simulink model "VGA_Interface"  (R2019b)
settings: Solver=VariableStepAuto  StartTime=0.0  StopTime=10.0  RelTol=1e-3
libraries: hdlsllib x24, simulink x20
settings Model: Creator=douglas.th  LastModifiedBy=Aaditya
settings DataIOCC: ReturnWorkspaceOutputs=off
settings OptimizationCC: BlockReduction=off  ConditionallyExecuteInputs=off  DefaultParameterBehavior=Inlined
settings DebuggingCC: AlgebraicLoopMsg=error  ArithmeticOperatorsInVariantConditions=warning
settings HardwareCC: ProdBitPerPointer=32  ProdBitPerSizeT=32  ProdBitPerPtrDiffT=32  ProdLargestAtomicFloat=None  ProdIntDivRoundTo=Undefined  ProdEndianess=Unspecified  ProdWordSize=32  ProdHWDeviceType=ASIC/FPGA->ASIC/FPGA  TargetBitPerPointer=64  TargetBitPerSizeT=64  TargetBitPerPtrDiffT=64  TargetLongLongMode=on  TargetIntDivRoundTo=Zero  TargetEndianess=LittleEndian  TargetWordSize=64  TargetHWDeviceType=Custom Processor->MATLAB Host Computer  ProdEqTarget=off
settings SFSimCC: SimUseLocalCustomCode=off  CustomCodeUndefinedFunction=UseInterfaceOnly
settings RTWCC: RTWUseLocalCustomCode=off

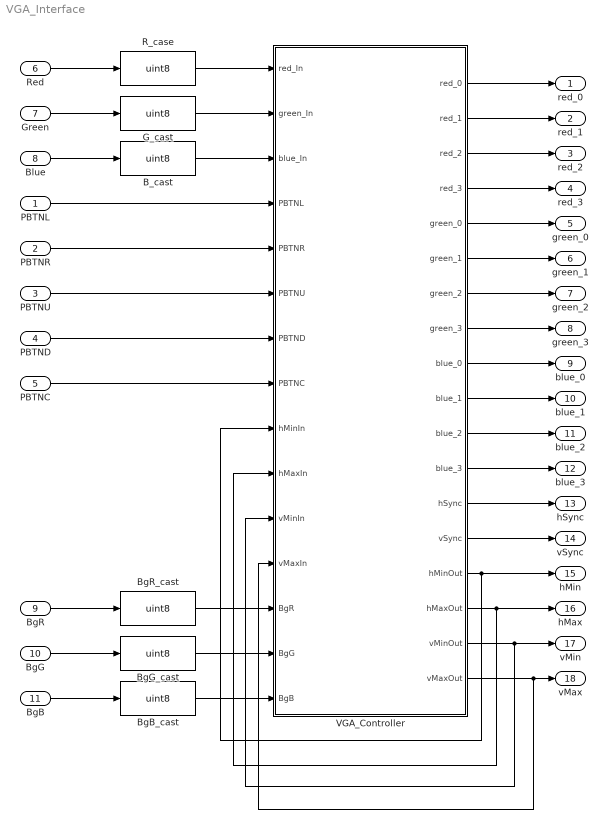
== system VGA_Interface ==
  PBTNL : Inport
  PBTNR : Inport  Port=2
  PBTNU : Inport  Port=3
  PBTND : Inport  Port=4
  PBTNC : Inport  Port=5
  Red : Inport  Port=6
  Green : Inport  Port=7
  Blue : Inport  Port=8
  BgR : Inport  Port=9
  BgG : Inport  Port=10
  BgB : Inport  Port=11
  B_cast : DataTypeConversion  OutDataTypeStr=uint8
  BgB_cast : DataTypeConversion  OutDataTypeStr=uint8
  BgG_cast : DataTypeConversion  OutDataTypeStr=uint8
  BgR_cast : DataTypeConversion  OutDataTypeStr=uint8
  G_cast : DataTypeConversion  OutDataTypeStr=uint8
  R_case : DataTypeConversion  OutDataTypeStr=uint8
  VGA_Controller : Subsystem
  red_0 : Outport  VectorParamsAs1DForOutWhenUnconnected=off
  red_1 : Outport  Port=2  VectorParamsAs1DForOutWhenUnconnected=off
  red_2 : Outport  Port=3  VectorParamsAs1DForOutWhenUnconnected=off
  red_3 : Outport  Port=4  VectorParamsAs1DForOutWhenUnconnected=off
  green_0 : Outport  Port=5  VectorParamsAs1DForOutWhenUnconnected=off
  green_1 : Outport  Port=6  VectorParamsAs1DForOutWhenUnconnected=off
  green_2 : Outport  Port=7  VectorParamsAs1DForOutWhenUnconnected=off
  green_3 : Outport  Port=8  VectorParamsAs1DForOutWhenUnconnected=off
  blue_0 : Outport  Port=9  VectorParamsAs1DForOutWhenUnconnected=off
  blue_1 : Outport  Port=10  VectorParamsAs1DForOutWhenUnconnected=off
  blue_2 : Outport  Port=11  VectorParamsAs1DForOutWhenUnconnected=off
  blue_3 : Outport  Port=12  VectorParamsAs1DForOutWhenUnconnected=off
  hSync : Outport  Port=13  VectorParamsAs1DForOutWhenUnconnected=off
  vSync : Outport  Port=14  VectorParamsAs1DForOutWhenUnconnected=off
  hMin : Outport  Port=15  VectorParamsAs1DForOutWhenUnconnected=off
  hMax : Outport  Port=16  VectorParamsAs1DForOutWhenUnconnected=off
  vMin : Outport  Port=17  VectorParamsAs1DForOutWhenUnconnected=off
  vMax : Outport  Port=18  VectorParamsAs1DForOutWhenUnconnected=off
  wires:
  VGA_Controller/1(red_0) -> red_0/1
  VGA_Controller/2(red_1) -> red_1/1
  VGA_Controller/3(red_2) -> red_2/1
  VGA_Controller/4(red_3) -> red_3/1
  VGA_Controller/5(green_0) -> green_0/1
  VGA_Controller/6(green_1) -> green_1/1
  VGA_Controller/7(green_2) -> green_2/1
  VGA_Controller/8(green_3) -> green_3/1
  VGA_Controller/9(blue_0) -> blue_0/1
  VGA_Controller/10(blue_1) -> blue_1/1
  VGA_Controller/11(blue_2) -> blue_2/1
  VGA_Controller/12(blue_3) -> blue_3/1
  VGA_Controller/14(vSync) -> vSync/1
  VGA_Controller/13(hSync) -> hSync/1
  Blue/1 -> B_cast/1
  G_cast/1 -> VGA_Controller/2(green_In)
  R_case/1 -> VGA_Controller/1(red_In)
  PBTNL/1 -> VGA_Controller/4(PBTNL)
  PBTNR/1 -> VGA_Controller/5(PBTNR)
  PBTNU/1 -> VGA_Controller/6(PBTNU)
  PBTND/1 -> VGA_Controller/7(PBTND)
  PBTNC/1 -> VGA_Controller/8(PBTNC)
  Red/1 -> R_case/1
  Green/1 -> G_cast/1
  B_cast/1 -> VGA_Controller/3(blue_In)
  VGA_Controller/16(hMaxOut) -> hMax/1, VGA_Controller/10(hMaxIn)
  VGA_Controller/15(hMinOut) -> VGA_Controller/9(hMinIn), hMin/1
  VGA_Controller/18(vMaxOut) -> VGA_Controller/12(vMaxIn), vMax/1
  VGA_Controller/17(vMinOut) -> vMin/1, VGA_Controller/11(vMinIn)
  BgB/1 -> BgB_cast/1
  BgB_cast/1 -> VGA_Controller/15(BgB)
  BgR/1 -> BgR_cast/1
  BgR_cast/1 -> VGA_Controller/13(BgR)
  BgG_cast/1 -> VGA_Controller/14(BgG)
  BgG/1 -> BgG_cast/1

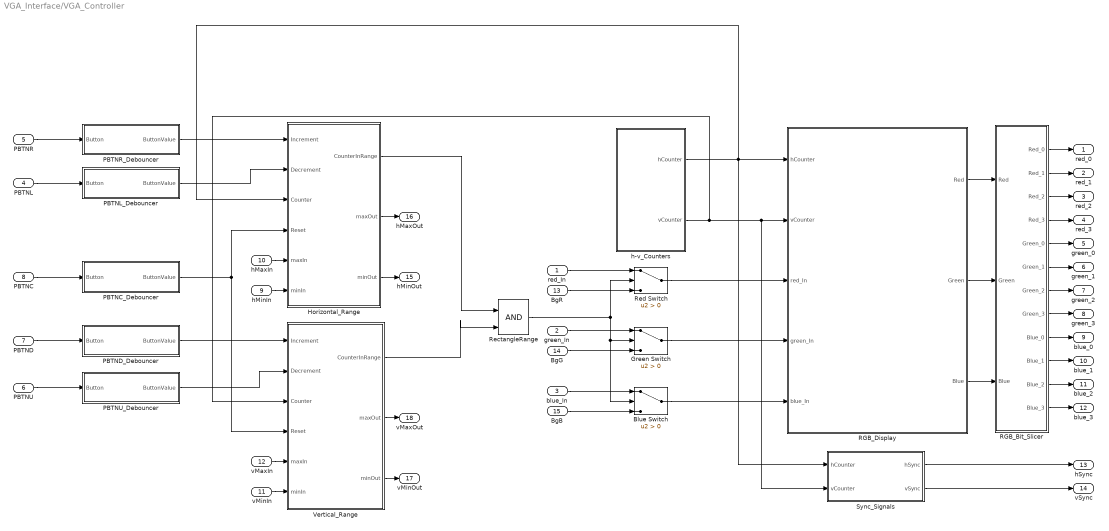
== system VGA_Interface/VGA_Controller ==
  red_In : Inport  OutDataTypeStr=uint8
  green_In : Inport  Port=2  OutDataTypeStr=uint8
  blue_In : Inport  Port=3  OutDataTypeStr=uint8
  PBTNL : Inport  Port=4  OutDataTypeStr=boolean
  PBTNR : Inport  Port=5  OutDataTypeStr=boolean
  PBTNU : Inport  Port=6  OutDataTypeStr=boolean
  PBTND : Inport  Port=7  OutDataTypeStr=boolean
  PBTNC : Inport  Port=8  OutDataTypeStr=boolean
  hMinIn : Inport  Port=9
  hMaxIn : Inport  Port=10
  vMinIn : Inport  Port=11
  vMaxIn : Inport  Port=12
  BgR : Inport  Port=13
  BgG : Inport  Port=14
  BgB : Inport  Port=15
  Blue Switch : Switch  Criteria=u2 > Threshold
  Green Switch : Switch  Criteria=u2 > Threshold
  Horizontal_Range : Subsystem
  PBTNC_Debouncer : Subsystem
  PBTND_Debouncer : Subsystem
  PBTNL_Debouncer : Subsystem
  PBTNR_Debouncer : Subsystem
  PBTNU_Debouncer : Subsystem
  RGB_Bit_Slicer : Subsystem
  RGB_Display : Subsystem
  RectangleRange : Logic  IconShape=distinctive  AllPortsSameDT=off  OutDataTypeStr=boolean
  Red Switch : Switch  Criteria=u2 > Threshold
  Sync_Signals : Subsystem
  Vertical_Range : Subsystem
  "h-v_Counters " : Subsystem
  red_0 : Outport  VectorParamsAs1DForOutWhenUnconnected=off
  red_1 : Outport  Port=2  VectorParamsAs1DForOutWhenUnconnected=off
  red_2 : Outport  Port=3  VectorParamsAs1DForOutWhenUnconnected=off
  red_3 : Outport  Port=4  VectorParamsAs1DForOutWhenUnconnected=off
  green_0 : Outport  Port=5  VectorParamsAs1DForOutWhenUnconnected=off
  green_1 : Outport  Port=6  VectorParamsAs1DForOutWhenUnconnected=off
  green_2 : Outport  Port=7  VectorParamsAs1DForOutWhenUnconnected=off
  green_3 : Outport  Port=8  VectorParamsAs1DForOutWhenUnconnected=off
  blue_0 : Outport  Port=9  VectorParamsAs1DForOutWhenUnconnected=off
  blue_1 : Outport  Port=10  VectorParamsAs1DForOutWhenUnconnected=off
  blue_2 : Outport  Port=11  VectorParamsAs1DForOutWhenUnconnected=off
  blue_3 : Outport  Port=12  VectorParamsAs1DForOutWhenUnconnected=off
  hSync : Outport  Port=13  VectorParamsAs1DForOutWhenUnconnected=off
  vSync : Outport  Port=14  VectorParamsAs1DForOutWhenUnconnected=off
  hMinOut : Outport  Port=15  VectorParamsAs1DForOutWhenUnconnected=off
  hMaxOut : Outport  Port=16  VectorParamsAs1DForOutWhenUnconnected=off
  vMinOut : Outport  Port=17  VectorParamsAs1DForOutWhenUnconnected=off
  vMaxOut : Outport  Port=18  VectorParamsAs1DForOutWhenUnconnected=off
  wires:
  RGB_Display/1(Red) -> RGB_Bit_Slicer/1(Red)
  RGB_Bit_Slicer/4(Red_3) -> red_3/1
  RGB_Display/2(Green) -> RGB_Bit_Slicer/2(Green)
  Sync_Signals/2(vSync) -> vSync/1
  RGB_Bit_Slicer/6(Green_1) -> green_1/1
  RGB_Bit_Slicer/1(Red_0) -> red_0/1
  RGB_Display/3(Blue) -> RGB_Bit_Slicer/3(Blue)
  Sync_Signals/1(hSync) -> hSync/1
  RGB_Bit_Slicer/3(Red_2) -> red_2/1
  RGB_Bit_Slicer/2(Red_1) -> red_1/1
  RGB_Bit_Slicer/5(Green_0) -> green_0/1
  RGB_Bit_Slicer/7(Green_2) -> green_2/1
  RGB_Bit_Slicer/8(Green_3) -> green_3/1
  RGB_Bit_Slicer/9(Blue_0) -> blue_0/1
  RGB_Bit_Slicer/10(Blue_1) -> blue_1/1
  RGB_Bit_Slicer/11(Blue_2) -> blue_2/1
  RGB_Bit_Slicer/12(Blue_3) -> blue_3/1
  red_In/1 -> Red Switch/1
  blue_In/1 -> Blue Switch/1
  green_In/1 -> Green Switch/1
  "h-v_Counters "/1(hCounter) -> RGB_Display/1(hCounter), Sync_Signals/1(hCounter), Horizontal_Range/3(Counter)
  Red Switch/1 -> RGB_Display/3(red_In)
  Green Switch/1 -> RGB_Display/4(green_In)
  Blue Switch/1 -> RGB_Display/5(blue_In)
  PBTNL/1 -> PBTNL_Debouncer/1(Button)
  PBTNR/1 -> PBTNR_Debouncer/1(Button)
  PBTNU/1 -> PBTNU_Debouncer/1(Button)
  PBTNC/1 -> PBTNC_Debouncer/1(Button)
  PBTNC_Debouncer/1(ButtonValue) -> Vertical_Range/4(Reset), Horizontal_Range/4(Reset)
  Horizontal_Range/1(CounterInRange) -> RectangleRange/1
  Vertical_Range/1(CounterInRange) -> RectangleRange/2
  RectangleRange/1 -> Red Switch/2, Blue Switch/2, Green Switch/2
  "h-v_Counters "/2(vCounter) -> Vertical_Range/3(Counter), RGB_Display/2(vCounter), Sync_Signals/2(vCounter)
  vMaxIn/1 -> Vertical_Range/5(maxIn)
  vMinIn/1 -> Vertical_Range/6(minIn)
  hMinIn/1 -> Horizontal_Range/6(minIn)
  hMaxIn/1 -> Horizontal_Range/5(maxIn)
  Horizontal_Range/3(minOut) -> hMinOut/1
  Horizontal_Range/2(maxOut) -> hMaxOut/1
  Vertical_Range/2(maxOut) -> vMaxOut/1
  Vertical_Range/3(minOut) -> vMinOut/1
  PBTNU_Debouncer/1(ButtonValue) -> Vertical_Range/2(Decrement)
  PBTNR_Debouncer/1(ButtonValue) -> Horizontal_Range/1(Increment)
  PBTNL_Debouncer/1(ButtonValue) -> Horizontal_Range/2(Decrement)
  PBTND_Debouncer/1(ButtonValue) -> Vertical_Range/1(Increment)
  PBTND/1 -> PBTND_Debouncer/1(Button)
  BgR/1 -> Red Switch/3
  BgG/1 -> Green Switch/3
  BgB/1 -> Blue Switch/3

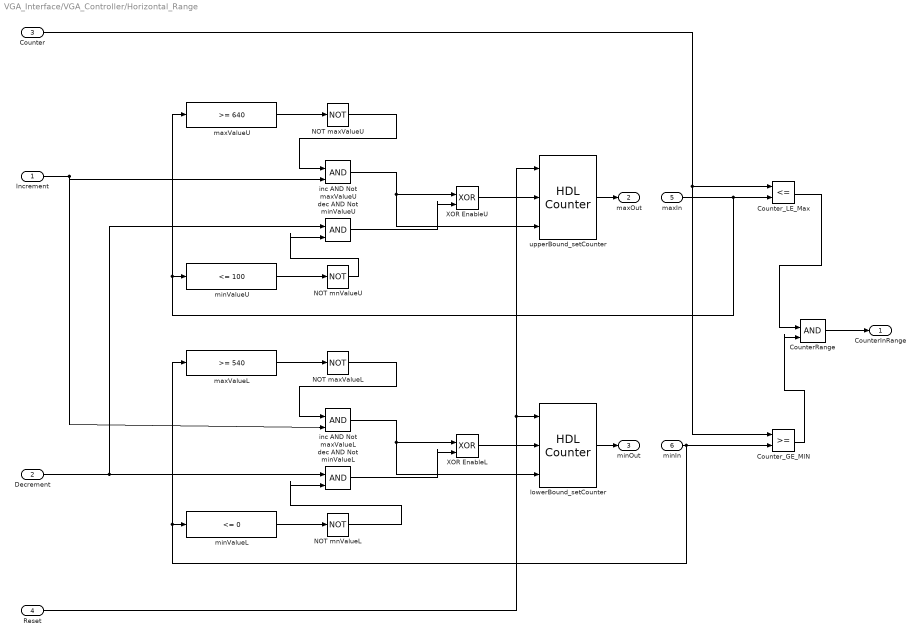
== system VGA_Interface/VGA_Controller/Horizontal_Range ==
  Increment : Inport
  Decrement : Inport  Port=2
  Counter : Inport  Port=3
  Reset : Inport  Port=4
  maxIn : Inport  Port=5  OutDataTypeStr=uint16
  minIn : Inport  Port=6  OutDataTypeStr=uint16
  CounterRange : Logic  IconShape=distinctive  AllPortsSameDT=off  OutDataTypeStr=boolean
  Counter_GE_MIN : RelationalOperator  OutDataTypeStr=boolean  RndMeth=Simplest
  Counter_LE_Max : RelationalOperator  Operator=<=  OutDataTypeStr=boolean  RndMeth=Simplest
  NOT maxValueL : Logic  Operator=NOT  IconShape=distinctive  AllPortsSameDT=off  OutDataTypeStr=boolean
  NOT maxValueU : Logic  Operator=NOT  IconShape=distinctive  AllPortsSameDT=off  OutDataTypeStr=boolean
  NOT mnValueL : Logic  Operator=NOT  IconShape=distinctive  AllPortsSameDT=off  OutDataTypeStr=boolean
  NOT mnValueU : Logic  Operator=NOT  IconShape=distinctive  AllPortsSameDT=off  OutDataTypeStr=boolean
  XOR EnableL : Logic  Operator=XOR  IconShape=distinctive  AllPortsSameDT=off  OutDataTypeStr=boolean
  XOR EnableU : Logic  Operator=XOR  IconShape=distinctive  AllPortsSameDT=off  OutDataTypeStr=boolean
  dec AND Not minValueL : Logic  IconShape=distinctive  AllPortsSameDT=off  OutDataTypeStr=boolean
  dec AND Not minValueU : Logic  IconShape=distinctive  AllPortsSameDT=off  OutDataTypeStr=boolean
  inc AND Not maxValueL : Logic  IconShape=distinctive  AllPortsSameDT=off  OutDataTypeStr=boolean
  inc AND Not maxValueU : Logic  IconShape=distinctive  AllPortsSameDT=off  OutDataTypeStr=boolean
  lowerBound_setCounter : hdlsllib/Sources/HDL Counter  CountType=Count limited  CountInit=0  CountStep=1  CountMax=540  CountFromType=Specify  CountFrom=0  CountResetPort=on  CountLoadPort=off  CountEnbPort=on  CountDirPort=on  CountDataType=Unsigned  CountWordLen=16  CountFracLen=0  CountSampTime=1
      settings: SourceProductBaseCode=HD
  maxValueL : simulink/Logic and Bit Operations/Compare To Constant  relop=>=  const=540  OutDataTypeStr=boolean
  maxValueU : simulink/Logic and Bit Operations/Compare To Constant  relop=>=  const=640  OutDataTypeStr=boolean
  minValueL : simulink/Logic and Bit Operations/Compare To Constant  relop=<=  const=0  OutDataTypeStr=boolean
  minValueU : simulink/Logic and Bit Operations/Compare To Constant  relop=<=  const=100  OutDataTypeStr=boolean
  upperBound_setCounter : hdlsllib/Sources/HDL Counter  CountType=Count limited  CountInit=100  CountStep=1  CountMax=640  CountFromType=Specify  CountFrom=100  CountResetPort=on  CountLoadPort=off  CountEnbPort=on  CountDirPort=on  CountDataType=Unsigned  CountWordLen=16  CountFracLen=0  CountSampTime=1
      settings: SourceProductBaseCode=HD
  CounterInRange : Outport  VectorParamsAs1DForOutWhenUnconnected=off
  maxOut : Outport  Port=2  OutDataTypeStr=uint16  VectorParamsAs1DForOutWhenUnconnected=off
  minOut : Outport  Port=3  OutDataTypeStr=uint16  VectorParamsAs1DForOutWhenUnconnected=off
  wires:
  inc AND Not maxValueU/1 -> XOR EnableU/1, upperBound_setCounter/3
  XOR EnableU/1 -> upperBound_setCounter/2
  minValueU/1 -> NOT mnValueU/1
  upperBound_setCounter/1 -> maxOut/1
  NOT maxValueU/1 -> inc AND Not maxValueU/1
  NOT mnValueU/1 -> dec AND Not minValueU/2
  maxValueU/1 -> NOT maxValueU/1
  dec AND Not minValueU/1 -> XOR EnableU/2
  Counter_LE_Max/1 -> CounterRange/1
  dec AND Not minValueL/1 -> XOR EnableL/2
  inc AND Not maxValueL/1 -> XOR EnableL/1, lowerBound_setCounter/3
  minValueL/1 -> NOT mnValueL/1
  NOT mnValueL/1 -> dec AND Not minValueL/2
  XOR EnableL/1 -> lowerBound_setCounter/2
  lowerBound_setCounter/1 -> minOut/1
  maxValueL/1 -> NOT maxValueL/1
  Counter/1 -> Counter_LE_Max/1, Counter_GE_MIN/1
  NOT maxValueL/1 -> inc AND Not maxValueL/1
  Counter_GE_MIN/1 -> CounterRange/2
  CounterRange/1 -> CounterInRange/1
  Decrement/1 -> dec AND Not minValueL/1, dec AND Not minValueU/1
  Increment/1 -> inc AND Not maxValueU/2, inc AND Not maxValueL/2
  Reset/1 -> upperBound_setCounter/1, lowerBound_setCounter/1
  maxIn/1 -> minValueU/1, maxValueU/1, Counter_LE_Max/2
  minIn/1 -> maxValueL/1, minValueL/1, Counter_GE_MIN/2

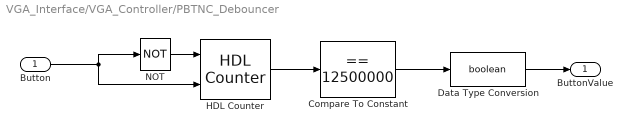
== system VGA_Interface/VGA_Controller/PBTNC_Debouncer ==
  Button : Inport
  Compare To Constant : simulink/Logic and Bit Operations/Compare To Constant  relop===  const=12500000  OutDataTypeStr=boolean
  Data Type Conversion : DataTypeConversion  OutDataTypeStr=boolean
  HDL Counter : hdlsllib/Sources/HDL Counter  CountType=Count limited  CountInit=0  CountStep=1  CountMax=50000000  CountFromType=Initial value  CountFrom=0  CountResetPort=on  CountLoadPort=off  CountEnbPort=on  CountDirPort=off  CountDataType=Unsigned  CountWordLen=32  CountFracLen=0  CountSampTime=1
      settings: SourceProductName=Simulink
  NOT : Logic  Operator=NOT  IconShape=distinctive  AllPortsSameDT=off  OutDataTypeStr=boolean
  ButtonValue : Outport  VectorParamsAs1DForOutWhenUnconnected=off
  wires:
  HDL Counter/1 -> Compare To Constant/1
  Compare To Constant/1 -> Data Type Conversion/1
  NOT/1 -> HDL Counter/1
  Button/1 -> HDL Counter/2, NOT/1
  Data Type Conversion/1 -> ButtonValue/1

== system VGA_Interface/VGA_Controller/PBTND_Debouncer ==
  Button : Inport
  Compare To Constant : simulink/Logic and Bit Operations/Compare To Constant  relop===  const=150000  OutDataTypeStr=boolean
  Data Type Conversion : DataTypeConversion  OutDataTypeStr=boolean
  HDL Counter : hdlsllib/Sources/HDL Counter  CountType=Count limited  CountInit=0  CountStep=1  CountMax=150000  CountFromType=Initial value  CountFrom=0  CountResetPort=on  CountLoadPort=off  CountEnbPort=on  CountDirPort=off  CountDataType=Unsigned  CountWordLen=32  CountFracLen=0  CountSampTime=1
      settings: SourceProductName=Simulink
  NOT : Logic  Operator=NOT  IconShape=distinctive  AllPortsSameDT=off  OutDataTypeStr=boolean
  ButtonValue : Outport  VectorParamsAs1DForOutWhenUnconnected=off
  wires:
  NOT/1 -> HDL Counter/1
  Button/1 -> HDL Counter/2, NOT/1
  Compare To Constant/1 -> Data Type Conversion/1
  HDL Counter/1 -> Compare To Constant/1
  Data Type Conversion/1 -> ButtonValue/1

== system VGA_Interface/VGA_Controller/PBTNL_Debouncer ==
  Button : Inport
  Compare To Constant : simulink/Logic and Bit Operations/Compare To Constant  relop===  const=150000  OutDataTypeStr=boolean
  Data Type Conversion : DataTypeConversion  OutDataTypeStr=boolean
  HDL Counter : hdlsllib/Sources/HDL Counter  CountType=Count limited  CountInit=0  CountStep=1  CountMax=150000  CountFromType=Initial value  CountFrom=0  CountResetPort=on  CountLoadPort=off  CountEnbPort=on  CountDirPort=off  CountDataType=Unsigned  CountWordLen=32  CountFracLen=0  CountSampTime=1
      settings: SourceProductName=Simulink
  NOT : Logic  Operator=NOT  IconShape=distinctive  AllPortsSameDT=off  OutDataTypeStr=boolean
  ButtonValue : Outport  VectorParamsAs1DForOutWhenUnconnected=off
  wires:
  NOT/1 -> HDL Counter/1
  Button/1 -> HDL Counter/2, NOT/1
  Compare To Constant/1 -> Data Type Conversion/1
  HDL Counter/1 -> Compare To Constant/1
  Data Type Conversion/1 -> ButtonValue/1

== system VGA_Interface/VGA_Controller/PBTNR_Debouncer ==
  Button : Inport
  Compare To Constant : simulink/Logic and Bit Operations/Compare To Constant  relop===  const=150000  OutDataTypeStr=boolean
  Data Type Conversion : DataTypeConversion  OutDataTypeStr=boolean
  HDL Counter : hdlsllib/Sources/HDL Counter  CountType=Count limited  CountInit=0  CountStep=1  CountMax=150000  CountFromType=Initial value  CountFrom=0  CountResetPort=on  CountLoadPort=off  CountEnbPort=on  CountDirPort=off  CountDataType=Unsigned  CountWordLen=32  CountFracLen=0  CountSampTime=1
      settings: SourceProductName=Simulink
  NOT : Logic  Operator=NOT  IconShape=distinctive  AllPortsSameDT=off  OutDataTypeStr=boolean
  ButtonValue : Outport  VectorParamsAs1DForOutWhenUnconnected=off
  wires:
  Button/1 -> HDL Counter/2, NOT/1
  Data Type Conversion/1 -> ButtonValue/1
  Compare To Constant/1 -> Data Type Conversion/1
  NOT/1 -> HDL Counter/1
  HDL Counter/1 -> Compare To Constant/1

== system VGA_Interface/VGA_Controller/PBTNU_Debouncer ==
  Button : Inport
  Compare To Constant : simulink/Logic and Bit Operations/Compare To Constant  relop===  const=150000  OutDataTypeStr=boolean
  Data Type Conversion : DataTypeConversion  OutDataTypeStr=boolean
  HDL Counter : hdlsllib/Sources/HDL Counter  CountType=Count limited  CountInit=0  CountStep=1  CountMax=150000  CountFromType=Initial value  CountFrom=0  CountResetPort=on  CountLoadPort=off  CountEnbPort=on  CountDirPort=off  CountDataType=Unsigned  CountWordLen=32  CountFracLen=0  CountSampTime=1
      settings: SourceProductName=Simulink
  NOT : Logic  Operator=NOT  IconShape=distinctive  AllPortsSameDT=off  OutDataTypeStr=boolean
  ButtonValue : Outport  VectorParamsAs1DForOutWhenUnconnected=off
  wires:
  NOT/1 -> HDL Counter/1
  Button/1 -> HDL Counter/2, NOT/1
  Compare To Constant/1 -> Data Type Conversion/1
  HDL Counter/1 -> Compare To Constant/1
  Data Type Conversion/1 -> ButtonValue/1

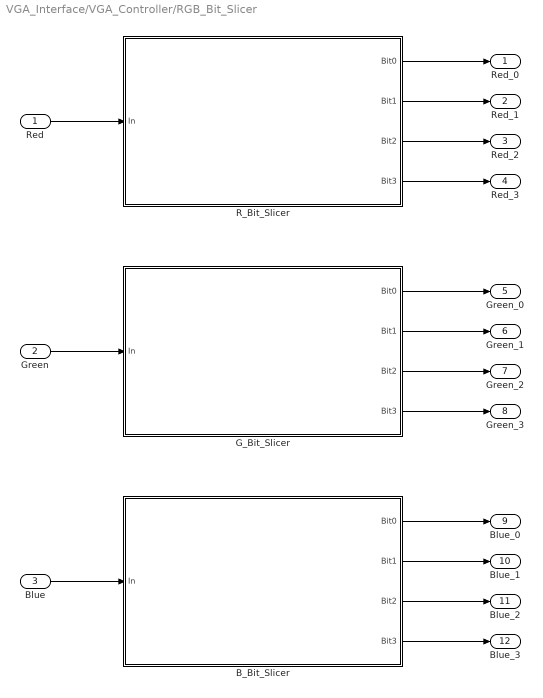
== system VGA_Interface/VGA_Controller/RGB_Bit_Slicer ==
  Red : Inport
  Green : Inport  Port=2
  Blue : Inport  Port=3
  B_Bit_Slicer : Subsystem
  G_Bit_Slicer : Subsystem
  R_Bit_Slicer : Subsystem
  Red_0 : Outport  VectorParamsAs1DForOutWhenUnconnected=off
  Red_1 : Outport  Port=2  VectorParamsAs1DForOutWhenUnconnected=off
  Red_2 : Outport  Port=3  VectorParamsAs1DForOutWhenUnconnected=off
  Red_3 : Outport  Port=4  VectorParamsAs1DForOutWhenUnconnected=off
  Green_0 : Outport  Port=5  VectorParamsAs1DForOutWhenUnconnected=off
  Green_1 : Outport  Port=6  VectorParamsAs1DForOutWhenUnconnected=off
  Green_2 : Outport  Port=7  VectorParamsAs1DForOutWhenUnconnected=off
  Green_3 : Outport  Port=8  VectorParamsAs1DForOutWhenUnconnected=off
  Blue_0 : Outport  Port=9  VectorParamsAs1DForOutWhenUnconnected=off
  Blue_1 : Outport  Port=10  VectorParamsAs1DForOutWhenUnconnected=off
  Blue_2 : Outport  Port=11  VectorParamsAs1DForOutWhenUnconnected=off
  Blue_3 : Outport  Port=12  VectorParamsAs1DForOutWhenUnconnected=off
  wires:
  Red/1 -> R_Bit_Slicer/1(In)
  R_Bit_Slicer/1(Bit0) -> Red_0/1
  R_Bit_Slicer/2(Bit1) -> Red_1/1
  R_Bit_Slicer/3(Bit2) -> Red_2/1
  R_Bit_Slicer/4(Bit3) -> Red_3/1
  Blue/1 -> B_Bit_Slicer/1(In)
  Green/1 -> G_Bit_Slicer/1(In)
  G_Bit_Slicer/1(Bit0) -> Green_0/1
  G_Bit_Slicer/4(Bit3) -> Green_3/1
  G_Bit_Slicer/3(Bit2) -> Green_2/1
  G_Bit_Slicer/2(Bit1) -> Green_1/1
  B_Bit_Slicer/1(Bit0) -> Blue_0/1
  B_Bit_Slicer/2(Bit1) -> Blue_1/1
  B_Bit_Slicer/3(Bit2) -> Blue_2/1
  B_Bit_Slicer/4(Bit3) -> Blue_3/1

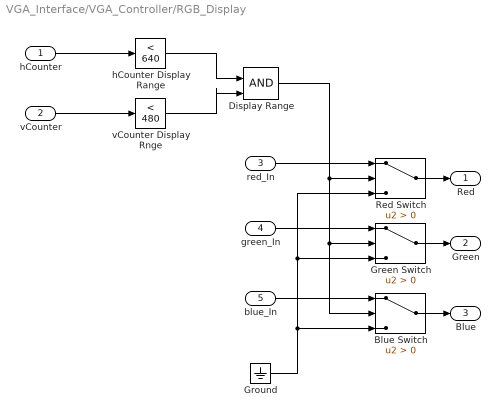
== system VGA_Interface/VGA_Controller/RGB_Display ==
  hCounter : Inport
  vCounter : Inport  Port=2
  red_In : Inport  Port=3  OutDataTypeStr=uint8
  green_In : Inport  Port=4  OutDataTypeStr=uint8
  blue_In : Inport  Port=5  OutDataTypeStr=uint8
  Blue Switch : Switch  Criteria=u2 > Threshold
  Display Range : Logic  IconShape=distinctive  AllPortsSameDT=off  OutDataTypeStr=boolean
  Green Switch : Switch  Criteria=u2 > Threshold
  Ground : Ground
  Red Switch : Switch  Criteria=u2 > Threshold
  hCounter Display Range : simulink/Logic and Bit Operations/Compare To Constant  relop=<  const=640  OutDataTypeStr=boolean
  vCounter Display Rnge : simulink/Logic and Bit Operations/Compare To Constant  relop=<  const=480  OutDataTypeStr=boolean
  Red : Outport  OutDataTypeStr=uint8  VectorParamsAs1DForOutWhenUnconnected=off
  Green : Outport  Port=2  OutDataTypeStr=uint8  VectorParamsAs1DForOutWhenUnconnected=off
  Blue : Outport  Port=3  OutDataTypeStr=uint8  VectorParamsAs1DForOutWhenUnconnected=off
  wires:
  blue_In/1 -> Blue Switch/1
  Blue Switch/1 -> Blue/1
  Ground/1 -> Blue Switch/3, Green Switch/3, Red Switch/3
  vCounter/1 -> vCounter Display Rnge/1
  hCounter/1 -> hCounter Display Range/1
  hCounter Display Range/1 -> Display Range/1
  vCounter Display Rnge/1 -> Display Range/2
  Red Switch/1 -> Red/1
  Green Switch/1 -> Green/1
  green_In/1 -> Green Switch/1
  red_In/1 -> Red Switch/1
  Display Range/1 -> Green Switch/2, Blue Switch/2, Red Switch/2

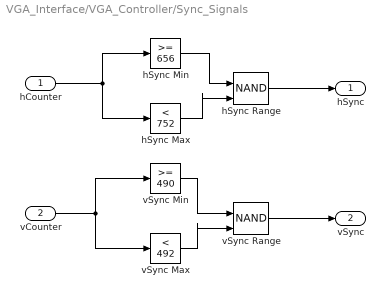
== system VGA_Interface/VGA_Controller/Sync_Signals ==
  hCounter : Inport
  vCounter : Inport  Port=2
  hSync Max : simulink/Logic and Bit Operations/Compare To Constant  relop=<  const=752  OutDataTypeStr=boolean
  hSync Min : simulink/Logic and Bit Operations/Compare To Constant  relop=>=  const=656  OutDataTypeStr=boolean
  hSync Range : Logic  Operator=NAND  IconShape=distinctive  AllPortsSameDT=off  OutDataTypeStr=boolean
  vSync Max : simulink/Logic and Bit Operations/Compare To Constant  relop=<  const=492  OutDataTypeStr=boolean
  vSync Min : simulink/Logic and Bit Operations/Compare To Constant  relop=>=  const=490  OutDataTypeStr=boolean
  vSync Range : Logic  Operator=NAND  IconShape=distinctive  AllPortsSameDT=off  OutDataTypeStr=boolean
  hSync : Outport  VectorParamsAs1DForOutWhenUnconnected=off
  vSync : Outport  Port=2  VectorParamsAs1DForOutWhenUnconnected=off
  wires:
  hSync Max/1 -> hSync Range/2
  hSync Min/1 -> hSync Range/1
  vSync Min/1 -> vSync Range/1
  vSync Max/1 -> vSync Range/2
  hCounter/1 -> hSync Max/1, hSync Min/1
  vCounter/1 -> vSync Max/1, vSync Min/1
  vSync Range/1 -> vSync/1
  hSync Range/1 -> hSync/1

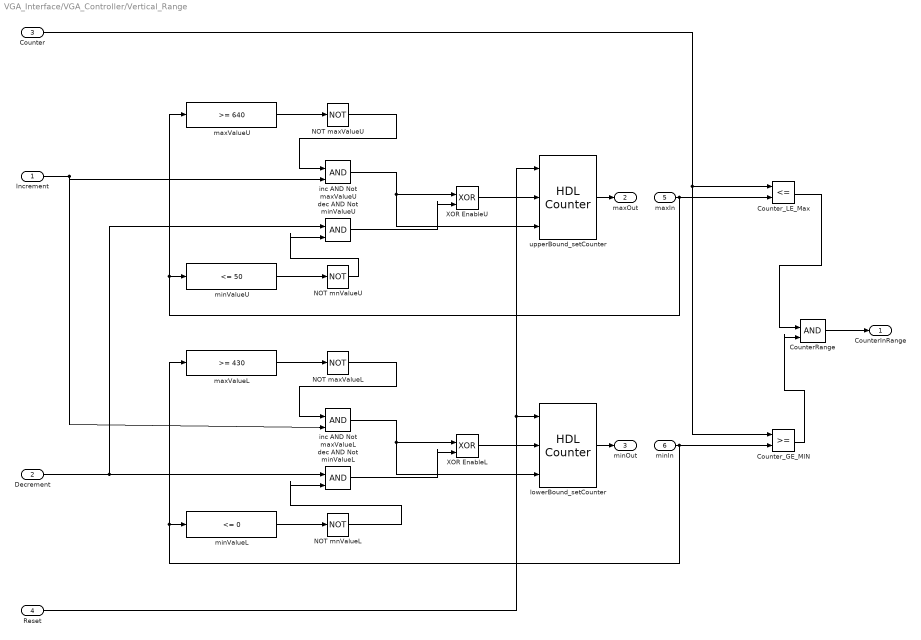
== system VGA_Interface/VGA_Controller/Vertical_Range ==
  Increment : Inport
  Decrement : Inport  Port=2
  Counter : Inport  Port=3
  Reset : Inport  Port=4
  maxIn : Inport  Port=5
  minIn : Inport  Port=6
  CounterRange : Logic  IconShape=distinctive  AllPortsSameDT=off  OutDataTypeStr=boolean
  Counter_GE_MIN : RelationalOperator  OutDataTypeStr=boolean  RndMeth=Simplest
  Counter_LE_Max : RelationalOperator  Operator=<=  OutDataTypeStr=boolean  RndMeth=Simplest
  NOT maxValueL : Logic  Operator=NOT  IconShape=distinctive  AllPortsSameDT=off  OutDataTypeStr=boolean
  NOT maxValueU : Logic  Operator=NOT  IconShape=distinctive  AllPortsSameDT=off  OutDataTypeStr=boolean
  NOT mnValueL : Logic  Operator=NOT  IconShape=distinctive  AllPortsSameDT=off  OutDataTypeStr=boolean
  NOT mnValueU : Logic  Operator=NOT  IconShape=distinctive  AllPortsSameDT=off  OutDataTypeStr=boolean
  XOR EnableL : Logic  Operator=XOR  IconShape=distinctive  AllPortsSameDT=off  OutDataTypeStr=boolean
  XOR EnableU : Logic  Operator=XOR  IconShape=distinctive  AllPortsSameDT=off  OutDataTypeStr=boolean
  dec AND Not minValueL : Logic  IconShape=distinctive  AllPortsSameDT=off  OutDataTypeStr=boolean
  dec AND Not minValueU : Logic  IconShape=distinctive  AllPortsSameDT=off  OutDataTypeStr=boolean
  inc AND Not maxValueL : Logic  IconShape=distinctive  AllPortsSameDT=off  OutDataTypeStr=boolean
  inc AND Not maxValueU : Logic  IconShape=distinctive  AllPortsSameDT=off  OutDataTypeStr=boolean
  lowerBound_setCounter : hdlsllib/Sources/HDL Counter  CountType=Count limited  CountInit=0  CountStep=1  CountMax=430  CountFromType=Specify  CountFrom=0  CountResetPort=on  CountLoadPort=off  CountEnbPort=on  CountDirPort=on  CountDataType=Unsigned  CountWordLen=16  CountFracLen=0  CountSampTime=1
      settings: SourceProductBaseCode=HD
  maxValueL : simulink/Logic and Bit Operations/Compare To Constant  relop=>=  const=430  OutDataTypeStr=boolean
  maxValueU : simulink/Logic and Bit Operations/Compare To Constant  relop=>=  const=640  OutDataTypeStr=boolean
  minValueL : simulink/Logic and Bit Operations/Compare To Constant  relop=<=  const=0  OutDataTypeStr=boolean
  minValueU : simulink/Logic and Bit Operations/Compare To Constant  relop=<=  const=50  OutDataTypeStr=boolean
  upperBound_setCounter : hdlsllib/Sources/HDL Counter  CountType=Count limited  CountInit=50  CountStep=1  CountMax=480  CountFromType=Specify  CountFrom=50  CountResetPort=on  CountLoadPort=off  CountEnbPort=on  CountDirPort=on  CountDataType=Unsigned  CountWordLen=16  CountFracLen=0  CountSampTime=1
      settings: SourceProductBaseCode=HD
  CounterInRange : Outport  VectorParamsAs1DForOutWhenUnconnected=off
  maxOut : Outport  Port=2  VectorParamsAs1DForOutWhenUnconnected=off
  minOut : Outport  Port=3  VectorParamsAs1DForOutWhenUnconnected=off
  wires:
  maxIn/1 -> maxValueU/1, minValueU/1, Counter_LE_Max/2
  minIn/1 -> maxValueL/1, minValueL/1, Counter_GE_MIN/2
  maxValueL/1 -> NOT maxValueL/1
  Reset/1 -> upperBound_setCounter/1, lowerBound_setCounter/1
  dec AND Not minValueU/1 -> XOR EnableU/2
  CounterRange/1 -> CounterInRange/1
  lowerBound_setCounter/1 -> minOut/1
  NOT maxValueL/1 -> inc AND Not maxValueL/1
  inc AND Not maxValueL/1 -> XOR EnableL/1, lowerBound_setCounter/3
  Counter/1 -> Counter_LE_Max/1, Counter_GE_MIN/1
  XOR EnableL/1 -> lowerBound_setCounter/2
  minValueL/1 -> NOT mnValueL/1
  Increment/1 -> inc AND Not maxValueU/2, inc AND Not maxValueL/2
  Counter_LE_Max/1 -> CounterRange/1
  minValueU/1 -> NOT mnValueU/1
  dec AND Not minValueL/1 -> XOR EnableL/2
  NOT mnValueL/1 -> dec AND Not minValueL/2
  NOT mnValueU/1 -> dec AND Not minValueU/2
  maxValueU/1 -> NOT maxValueU/1
  Decrement/1 -> dec AND Not minValueL/1, dec AND Not minValueU/1
  NOT maxValueU/1 -> inc AND Not maxValueU/1
  inc AND Not maxValueU/1 -> XOR EnableU/1, upperBound_setCounter/3
  XOR EnableU/1 -> upperBound_setCounter/2
  Counter_GE_MIN/1 -> CounterRange/2
  upperBound_setCounter/1 -> maxOut/1

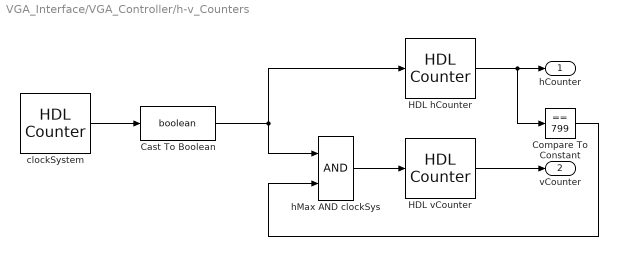
== system VGA_Interface/VGA_Controller/h-v_Counters  ==
  Cast To Boolean : DataTypeConversion  OutDataTypeStr=boolean
  Compare To Constant : simulink/Logic and Bit Operations/Compare To Constant  relop===  const=799  OutDataTypeStr=boolean
  HDL hCounter : hdlsllib/Sources/HDL Counter  CountType=Count limited  CountInit=0  CountStep=1  CountMax=799  CountFromType=Initial value  CountFrom=0  CountResetPort=off  CountLoadPort=off  CountEnbPort=on  CountDirPort=off  CountDataType=Unsigned  CountWordLen=10  CountFracLen=0  CountSampTime=1
      settings: SourceProductBaseCode=HD
  "HDL vCounter " : hdlsllib/Sources/HDL Counter  CountType=Count limited  CountInit=0  CountStep=1  CountMax=524  CountFromType=Initial value  CountFrom=0  CountResetPort=off  CountLoadPort=off  CountEnbPort=on  CountDirPort=off  CountDataType=Unsigned  CountWordLen=10  CountFracLen=0  CountSampTime=1
      settings: SourceProductBaseCode=HD
  clockSystem : hdlsllib/Sources/HDL Counter  CountType=Free running  CountInit=1  CountStep=1  CountMax=25  CountFromType=Initial value  CountFrom=1  CountResetPort=off  CountLoadPort=off  CountEnbPort=off  CountDirPort=off  CountDataType=Unsigned  CountWordLen=1  CountFracLen=0  CountSampTime=1
      settings: SourceProductBaseCode=HD
  hMax AND clockSys : Logic  IconShape=distinctive  AllPortsSameDT=off  OutDataTypeStr=boolean
  hCounter : Outport  VectorParamsAs1DForOutWhenUnconnected=off
  vCounter : Outport  Port=2  VectorParamsAs1DForOutWhenUnconnected=off
  wires:
  "HDL vCounter "/1 -> vCounter/1
  clockSystem/1 -> Cast To Boolean/1
  HDL hCounter/1 -> Compare To Constant/1, hCounter/1
  hMax AND clockSys/1 -> "HDL vCounter "/1
  Compare To Constant/1 -> hMax AND clockSys/2
  Cast To Boolean/1 -> HDL hCounter/1, hMax AND clockSys/1

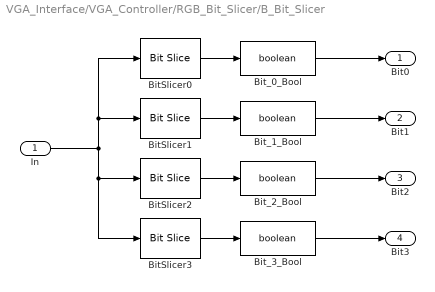
== system VGA_Interface/VGA_Controller/RGB_Bit_Slicer/B_Bit_Slicer ==
  In : Inport
  BitSlicer0 : hdlsllib/Logic and Bit Operations/Bit Slice  lidx=0  ridx=0
  BitSlicer1 : hdlsllib/Logic and Bit Operations/Bit Slice  lidx=1  ridx=1
  BitSlicer2 : hdlsllib/Logic and Bit Operations/Bit Slice  lidx=2  ridx=2
  BitSlicer3 : hdlsllib/Logic and Bit Operations/Bit Slice  lidx=3  ridx=3
  Bit_0_Bool : DataTypeConversion  OutDataTypeStr=boolean
  Bit_1_Bool : DataTypeConversion  OutDataTypeStr=boolean
  Bit_2_Bool : DataTypeConversion  OutDataTypeStr=boolean
  Bit_3_Bool : DataTypeConversion  OutDataTypeStr=boolean
  Bit0 : Outport  VectorParamsAs1DForOutWhenUnconnected=off
  Bit1 : Outport  Port=2  VectorParamsAs1DForOutWhenUnconnected=off
  Bit2 : Outport  Port=3  VectorParamsAs1DForOutWhenUnconnected=off
  Bit3 : Outport  Port=4  VectorParamsAs1DForOutWhenUnconnected=off
  wires:
  Bit_1_Bool/1 -> Bit1/1
  BitSlicer2/1 -> Bit_2_Bool/1
  Bit_3_Bool/1 -> Bit3/1
  Bit_2_Bool/1 -> Bit2/1
  In/1 -> BitSlicer3/1, BitSlicer2/1, BitSlicer0/1, BitSlicer1/1
  BitSlicer3/1 -> Bit_3_Bool/1
  Bit_0_Bool/1 -> Bit0/1
  BitSlicer0/1 -> Bit_0_Bool/1
  BitSlicer1/1 -> Bit_1_Bool/1

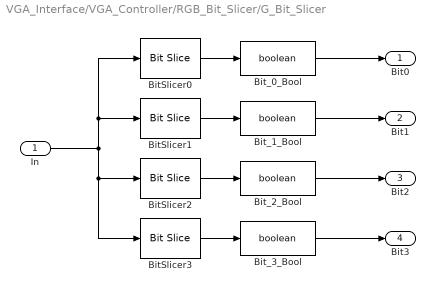
== system VGA_Interface/VGA_Controller/RGB_Bit_Slicer/G_Bit_Slicer ==
  In : Inport
  BitSlicer0 : hdlsllib/Logic and Bit Operations/Bit Slice  lidx=0  ridx=0
  BitSlicer1 : hdlsllib/Logic and Bit Operations/Bit Slice  lidx=1  ridx=1
  BitSlicer2 : hdlsllib/Logic and Bit Operations/Bit Slice  lidx=2  ridx=2
  BitSlicer3 : hdlsllib/Logic and Bit Operations/Bit Slice  lidx=3  ridx=3
  Bit_0_Bool : DataTypeConversion  OutDataTypeStr=boolean
  Bit_1_Bool : DataTypeConversion  OutDataTypeStr=boolean
  Bit_2_Bool : DataTypeConversion  OutDataTypeStr=boolean
  Bit_3_Bool : DataTypeConversion  OutDataTypeStr=boolean
  Bit0 : Outport  VectorParamsAs1DForOutWhenUnconnected=off
  Bit1 : Outport  Port=2  VectorParamsAs1DForOutWhenUnconnected=off
  Bit2 : Outport  Port=3  VectorParamsAs1DForOutWhenUnconnected=off
  Bit3 : Outport  Port=4  VectorParamsAs1DForOutWhenUnconnected=off
  wires:
  Bit_1_Bool/1 -> Bit1/1
  BitSlicer2/1 -> Bit_2_Bool/1
  Bit_3_Bool/1 -> Bit3/1
  Bit_2_Bool/1 -> Bit2/1
  In/1 -> BitSlicer3/1, BitSlicer2/1, BitSlicer0/1, BitSlicer1/1
  BitSlicer3/1 -> Bit_3_Bool/1
  Bit_0_Bool/1 -> Bit0/1
  BitSlicer0/1 -> Bit_0_Bool/1
  BitSlicer1/1 -> Bit_1_Bool/1

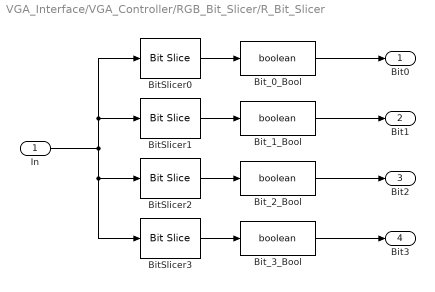
== system VGA_Interface/VGA_Controller/RGB_Bit_Slicer/R_Bit_Slicer ==
  In : Inport
  BitSlicer0 : hdlsllib/Logic and Bit Operations/Bit Slice  lidx=0  ridx=0
  BitSlicer1 : hdlsllib/Logic and Bit Operations/Bit Slice  lidx=1  ridx=1
  BitSlicer2 : hdlsllib/Logic and Bit Operations/Bit Slice  lidx=2  ridx=2
  BitSlicer3 : hdlsllib/Logic and Bit Operations/Bit Slice  lidx=3  ridx=3
  Bit_0_Bool : DataTypeConversion  OutDataTypeStr=boolean
  Bit_1_Bool : DataTypeConversion  OutDataTypeStr=boolean
  Bit_2_Bool : DataTypeConversion  OutDataTypeStr=boolean
  Bit_3_Bool : DataTypeConversion  OutDataTypeStr=boolean
  Bit0 : Outport  VectorParamsAs1DForOutWhenUnconnected=off
  Bit1 : Outport  Port=2  VectorParamsAs1DForOutWhenUnconnected=off
  Bit2 : Outport  Port=3  VectorParamsAs1DForOutWhenUnconnected=off
  Bit3 : Outport  Port=4  VectorParamsAs1DForOutWhenUnconnected=off
  wires:
  Bit_1_Bool/1 -> Bit1/1
  BitSlicer2/1 -> Bit_2_Bool/1
  Bit_3_Bool/1 -> Bit3/1
  Bit_2_Bool/1 -> Bit2/1
  In/1 -> BitSlicer3/1, BitSlicer2/1, BitSlicer0/1, BitSlicer1/1
  BitSlicer3/1 -> Bit_3_Bool/1
  Bit_0_Bool/1 -> Bit0/1
  BitSlicer0/1 -> Bit_0_Bool/1
  BitSlicer1/1 -> Bit_1_Bool/1
